simulink model "etc_PI_singletasking"  (R2018a)
settings: Solver=FixedStepDiscrete  StartTime=0.0  StopTime=2.5  RelTol=1e-3
PreLoadFcn:
  | Ki = 2;
  | Kp = 0.3;
  | Ts = 0.01;
settings Model: Creator=jrivitus  LastModifiedBy=bneiswan
settings DataIOCC: LimitDataPoints=on  SaveFormat=Array
settings OptimizationCC: ExpressionDepthLimit=2147483647  InitFltsAndDblsToZero=on  LifeSpan=1
settings DebuggingCC: UnderspecifiedInitializationDetection=Classic  MergeDetectMultiDrivingBlocksExec=none  ParameterPrecisionLossMsg=none  FcnCallInpInsideContextMsg=warning  AllowSymbolicDim=off  StateNameClashWarn=warning  SFUnexpectedBacktrackingDiag=warning  SFNoUnconditionalDefaultTransitionDiag=warning  SFExecutionAtInitializationDiag=none
settings HardwareCC: ProdBitPerPointer=32  ProdBitPerSizeT=32  ProdBitPerPtrDiffT=32  ProdLargestAtomicFloat=None  ProdIntDivRoundTo=Undefined  ProdEndianess=Unspecified  ProdWordSize=32  ProdHWDeviceType=32-bit Generic
settings ModelReferenceCC: PropagateSignalLabelsOutOfModel=off
settings SFSimCC: MATLABDynamicMemAlloc=off
settings RTWCC: SystemTargetFile=ert.tlc  GenCodeOnly=on  TemplateMakefile=ert_default_tmf  Description=Real-Time Workshop Embedded Coder (no auto configuration)  GenerateReport=on  IncludeHyperlinkInReport=on  LaunchReport=on  GenerateTraceInfo=on
settings CodeAppCC: IgnoreCustomStorageClasses=off  CustomSymbolStrType=$N$R$M  StateflowObjectComments=on  InternalIdentifier=Classic
settings ERTTargetCC: MultiwordLength=2048  GenerateSampleERTMain=on  SupportContinuousTime=on  ERTCustomFileTemplate=example_file_process.tlc  ConvertIfToSwitch=off  SuppressUnreachableDefaultCases=off
settings ConfigComp: CovMetricSettings=dw  CovHtmlReporting=on  CovSaveCumulativeToWorkspaceVar=on  CovSaveSingleToWorkspaceVar=on  CovExternalEMLEnable=off  CovSFcnEnable=off

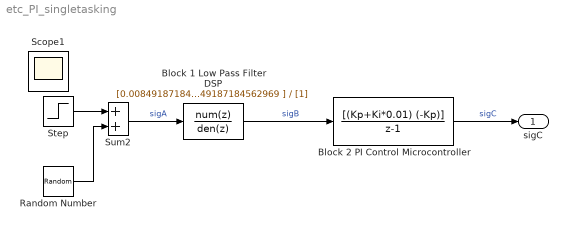
== system etc_PI_singletasking ==
  Block 1 Low Pass Filter DSP : DiscreteFilter  Numerator=|  Denominator=[1]  SampleTime=0.005
      | [0.00849187184562969	0.0444846983267221	0.117299133563462	0.199122538167043	0.235872521380986	0.199122538167043	0.117299133563462	0.0444846983267221	0.00849187184562969
      | ]
      settings: AttributesFormatString=Ts = %<SampleTime>
  Block 2 PI Control Microcontroller : DiscreteTransferFcn  Numerator=[(Kp+Ki*0.01) (-Kp)]  Denominator=[1 -1]  SampleTime=0.01
      settings: AttributesFormatString=Ts = %<SampleTime>
  Random Number : RandomNumber  Variance=0.01  SampleTime=0.005
      settings: AttributesFormatString=Mean: %<Mean>\nVariance: %<Variance>
  Step : Step  SampleTime=0.005
  Sum2 : Sum  SaturateOnIntegerOverflow=on  InputSameDT=on  OutDataTypeStr=Inherit: Same as first input
  sigC : Outport
  Scope1 : Scope
  wires:
  Sum2/1 -> Block 1 Low Pass Filter DSP/1  "sigA"
  Step/1 -> Sum2/1
  Random Number/1 -> Sum2/2
  Block 2 PI Control Microcontroller/1 -> sigC/1  "sigC"
  Block 1 Low Pass Filter DSP/1 -> Block 2 PI Control Microcontroller/1  "sigB"
